simulink model "LinearSimulationarmonly"  (R2017a)
settings: Solver=VariableStepAuto  StartTime=0.0  StopTime=5  RelTol=1e-3
libraries: simulink x3
settings Model: Creator=khrom  LastModifiedBy=khrom

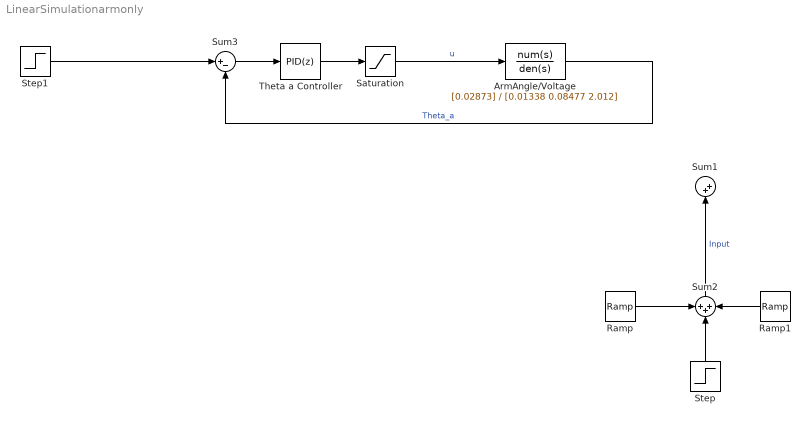
== system LinearSimulationarmonly ==
  ArmAngle/Voltage : TransferFcn  Numerator=[0.02873]  Denominator=[0.01338 0.08477 2.012]
  Ramp : simulink/Sources/Ramp  slope=sin(pi/180)  start=0  X0=0
  Ramp1 : simulink/Sources/Ramp  slope=-sin(pi/180)  start=0.1  X0=0
  Saturation : Saturate  UpperLimit=14  LowerLimit=-14
  Step : Step  Time=0.1  After=-sin(2*pi/180)*0.1  SampleTime=0
  Step1 : Step  Time=0  After=sin(5*pi/180)  SampleTime=0
  Sum1 : Sum  Inputs=|++
  Sum2 : Sum  Inputs=+++
  Sum3 : Sum  Inputs=|+-
  Theta a Controller : simulink/Continuous/PID Controller  Controller=PID  TimeDomain=Discrete-time  SampleTime=1e-3  IntegratorMethod=Forward Euler  FilterMethod=Forward Euler  Form=Parallel  UseFilter=on  ControllerParametersSource=internal  P=400  I=900  D=25  N=100  InitialConditionSource=internal  InitialConditionForIntegrator=0  InitialConditionForFilter=0  ExternalReset=none  LimitOutput=off  UpperSaturationLimit=inf  LowerSaturationLimit=-inf  LinearizeAsGain=off  AntiWindupMode=none  Kb=1  TrackingMode=off  Kt=1  PParamMin=[]  PParamMax=[]  IParamMin=[]  IParamMax=[]  DParamMin=[]  DParamMax=[]  NParamMin=[]  NParamMax=[]  KbParamMin=[]  KbParamMax=[]  KtParamMin=[]  KtParamMax=[]  POutMin=[]  POutMax=[]  IOutMin=[]  IOutMax=[]  DOutMin=[]  DOutMax=[]  NOutMin=[]  NOutMax=[]  KbOutMin=[]  KbOutMax=[]  KtOutMin=[]  KtOutMax=[]  IntegratorOutMin=[]  IntegratorOutMax=[]  FilterOutMin=[]  FilterOutMax=[]  SumOutMin=[]  SumOutMax=[]  SumI1OutMin=[]  SumI1OutMax=[]  SumI2OutMin=[]  SumI2OutMax=[]  SumI3OutMin=[]  SumI3OutMax=[]  SumDOutMin=[]  SumDOutMax=[]  SaturationOutMin=[]  SaturationOutMax=[]  IntegratorContinuousStateAttributes=''  IntegratorStateMustResolveToSignalObject=off  IntegratorRTWStateStorageClass=Auto  FilterContinuousStateAttributes=''  FilterStateMustResolveToSignalObject=off  FilterRTWStateStorageClass=Auto  DifferentiatorICPrevScaledInput=0  DifferentiatorOutMin=[]  DifferentiatorOutMax=[]  InitialConditionSetting=State (most efficient)
  wires:
  Sum3/1 -> Theta a Controller/1
  ArmAngle/Voltage/1 -> Sum3/2  "Theta_a"
  Sum2/1 -> Sum1/2  "Input"
  Theta a Controller/1 -> Saturation/1
  Ramp/1 -> Sum2/1
  Ramp1/1 -> Sum2/3
  Step/1 -> Sum2/2
  Step1/1 -> Sum3/1
  Saturation/1 -> ArmAngle/Voltage/1  "u"
